simulink library "fc_vt_lib"  (Simulink 4.00)
undefined symbols (not defined in the file or in its folder): amb_tmp, compressor_mass_flow_map, compressor_pressure_map, compressor_temperature_rise_map, fc_air_comp_scale, fc_allowable_temp_rise, fc_cathode_pressure_drop, fc_cell_area, fc_cell_num, fc_comp_adeff_max, fc_comp_elec_eff, fc_comp_max_tmp, fc_comp_slpm_air_max, fc_comp_spd_max, fc_comp_voleff_max, fc_condenser_fan_flowrate, fc_condenser_fan_num, fc_condenser_fan_pwr_map, fc_condenser_frontal_area, fc_condenser_scale, fc_coolant_pump_flow_map, fc_coolant_pump_pwr_map, fc_cp_air, fc_cp_h2o_l, fc_cp_stack, fc_fuel_lhv, fc_k_air, fc_max_cathode_inlet_pressure, fc_min_cathode_inlet_pressure, fc_min_cell_volts, fc_min_sys_pwr_req, fc_min_temp_for_heat_rejection, fc_mw_air, fc_mw_h2, fc_mw_h20, fc_o2_percent, fc_p_amb, fc_polar_param_concentration, fc_polar_param_ohmic, fc_polar_param_ohmic_temp, fc_polar_param_ref_temp, fc_polar_param_tafel, fc_polar_param_temperature, fc_polar_param_voc, fc_radiator_bypass_delta_t, fc_radiator_fan_flowrate, fc_radiator_fan_num, fc_radiator_fan_pwr_map, fc_radiator_frontal_area, fc_radiator_no_fan_flowrate, fc_radiator_scale, fc_radiator_spd_ratio_fan_off, fc_radiator_spd_ratio_fan_on, fc_radiator_veh_spd_map, fc_reference_temperature, fc_rh_amb, fc_stack_i_map, fc_stack_pres_cor_map, fc_stack_pres_map, fc_stack_stoich_air_map ... (+10)
libraries: fc_vt_lib x54, simulink3 x9
(part 1 of 3)
settings Model: LastModifiedBy=kharalds

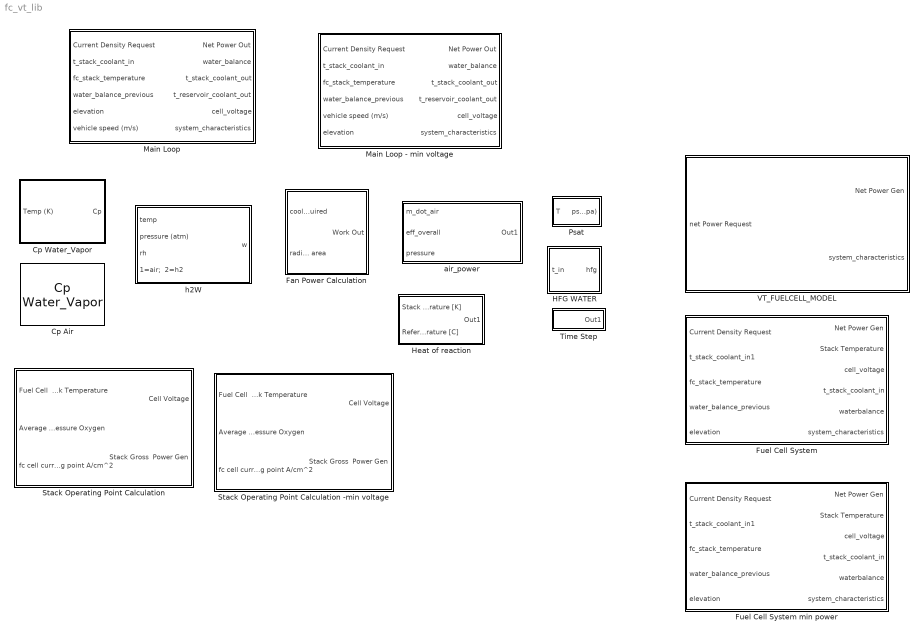
== system fc_vt_lib ==
  Cp Air : fc_vt_lib/Cp Water_Vapor
      settings: RTWFcnNameOpts=Auto  RTWFileNameOpts=Auto
  Cp Water_Vapor : Subsystem
      settings: RTWFcnNameOpts=Auto  RTWFileNameOpts=Auto
  Fan Power Calculation : Subsystem
      settings: RTWFcnNameOpts=Auto  RTWFileNameOpts=Auto
  Fuel Cell System : Subsystem
      settings: RTWFcnNameOpts=Auto  RTWFileNameOpts=Auto
  Fuel Cell System min power : Subsystem
      settings: RTWFcnNameOpts=Auto  RTWFileNameOpts=Auto
  HFG WATER : Subsystem
      settings: RTWFcnNameOpts=Auto  RTWFileNameOpts=Auto
  Heat of reaction : Subsystem
      settings: RTWFcnNameOpts=Auto  RTWFileNameOpts=Auto
  Main Loop : Subsystem
      settings: RTWFcnNameOpts=Auto  RTWFileNameOpts=Auto
  Main Loop - min voltage : Subsystem
      settings: RTWFcnNameOpts=Auto  RTWFileNameOpts=Auto
  Psat : Subsystem
      settings: RTWFcnNameOpts=Auto  RTWFileNameOpts=Auto
  Stack Operating Point Calculation : Subsystem
      settings: RTWFcnNameOpts=Auto  RTWFileNameOpts=Auto
  Stack Operating Point Calculation -min voltage : Subsystem
      settings: RTWFcnNameOpts=Auto  RTWFileNameOpts=Auto
  Time Step : Subsystem
      settings: RTWFcnNameOpts=Auto  RTWFileNameOpts=Auto
  VT_FUELCELL_MODEL : Subsystem
      settings: RTWFcnNameOpts=Auto  RTWFileNameOpts=Auto
  air_power : Subsystem
      settings: RTWFcnNameOpts=Auto  RTWFileNameOpts=Auto
  h2W : Subsystem
      settings: RTWFcnNameOpts=Auto  RTWFileNameOpts=Auto

== system fc_vt_lib/Cp Water_Vapor ==
  Temp (K) : Inport  Port=1  LatchInput=off
  A : Constant  Value=32.24
  B : Constant  Value=.1923E-2
  C : Constant  Value=1.055E-5
  D : Constant  Value=-3.595E-9
  D1 : Constant  Value=3
  D2 : Constant  Value=2
  Gain : Gain  Gain=1000  Multiplication=Element-wise(K.*u)  SaturateOnIntegerOverflow=on
  Gain1 : Gain  Gain=1/18.015  Multiplication=Element-wise(K.*u)  SaturateOnIntegerOverflow=on
  Math Function : Math  Operator=pow  OutputSignalType=auto
  Math Function1 : Math  Operator=pow  OutputSignalType=auto
  Product : Product  Inputs=2  Multiplication=Element-wise(.*)  SaturateOnIntegerOverflow=on
  Product1 : Product  Inputs=2  Multiplication=Element-wise(.*)  SaturateOnIntegerOverflow=on
  Product2 : Product  Inputs=2  Multiplication=Element-wise(.*)  SaturateOnIntegerOverflow=on
  Sum : Sum  Inputs=++++  SaturateOnIntegerOverflow=on
  Cp : Outport  Port=1
  wires:
  A/1 -> Sum/1
  B/1 -> Product/2
  Product/1 -> Sum/2
  Math Function/1 -> Product1/1
  C/1 -> Product1/2
  Math Function1/1 -> Product2/1
  D/1 -> Product2/2
  D1/1 -> Math Function1/2
  D2/1 -> Math Function/2
  Temp (K)/1 -> Math Function1/1, Math Function/1, Product/1
  Product1/1 -> Sum/3
  Product2/1 -> Sum/4
  Sum/1 -> Gain/1
  Gain/1 -> Gain1/1
  Gain1/1 -> Cp/1

== system fc_vt_lib/Fan Power Calculation ==
  cooling air  required : Inport  Port=1  LatchInput=off
  radiator frontal area : Inport  Port=2  LatchInput=off
  Constant : Constant  Value=273.15
  Constant2 : Constant  Value=fc_cp_air
  Math Function : Math  Operator=pow  OutputSignalType=auto
  Pressure Drop Relation massflow (kg/s)->Pa : Fcn  Expr=(326.21*u(1)-75.396)+101325
  Product2 : Product  Inputs=*/  Multiplication=Element-wise(.*)  SaturateOnIntegerOverflow=on
  Sum : Sum  Inputs=|++  SaturateOnIntegerOverflow=on
  Sum2 : Sum  Inputs=-+  SaturateOnIntegerOverflow=on
  Sum3 : Sum  Inputs=-+  SaturateOnIntegerOverflow=on
  T_amb1 : Constant  Value=fc_k_air
  T_amb2 : Constant  Value=1
  Work Fan  Temperature  Difference Calc1 : Product  Inputs=*/  Multiplication=Element-wise(.*)  SaturateOnIntegerOverflow=on
  Work Fan Calc : Product  Inputs=****/  Multiplication=Element-wise(.*)  SaturateOnIntegerOverflow=on
  ambient temp (C) : Constant  Value=amb_tmp
  leave it alone!4 : Constant  Value=101325
  Work Out : Outport  Port=1
  wires:
  Constant2/1 -> Work Fan Calc/3
  Sum2/1 -> Work Fan  Temperature  Difference Calc1/1
  T_amb2/1 -> Sum2/1, Sum3/1
  T_amb1/1 -> Sum2/2, Work Fan  Temperature  Difference Calc1/2
  Pressure Drop Relation massflow (kg/s)->Pa/1 -> Product2/1
  leave it alone!4/1 -> Product2/2
  Product2/1 -> Math Function/1
  cooling air  required/1 -> Work Fan Calc/2, Pressure Drop Relation massflow (kg/s)->Pa/1
  radiator frontal area/1 -> Work Fan Calc/5
  Work Fan Calc/1 -> Work Out/1
  Math Function/1 -> Sum3/2
  Work Fan  Temperature  Difference Calc1/1 -> Math Function/2
  Sum3/1 -> Work Fan Calc/1
  Sum/1 -> Work Fan Calc/4
  Constant/1 -> Sum/1
  ambient temp (C)/1 -> Sum/2

== system fc_vt_lib/Fuel Cell System ==
  " Current Density Request" : Inport  Port=1  LatchInput=off
  t_stack_coolant_in1 : Inport  Port=2  LatchInput=off
  fc_stack_temperature : Inport  Port=3  LatchInput=off
  water_balance_previous : Inport  Port=4  LatchInput=off
  elevation : Inport  Port=5  LatchInput=off
  Main Loop : fc_vt_lib/Main Loop
      settings: RTWFcnNameOpts=Auto  RTWFileNameOpts=Auto
  Net Power Gen : Outport  Port=1
  Stack Temperature : Outport  Port=2
  cell_voltage : Outport  Port=3
  t_stack_coolant_in : Outport  Port=4
  waterbalance : Outport  Port=5
  system_characteristics : Outport  Port=6
  wires:
  Main Loop/1 -> Net Power Gen/1
  Main Loop/4 -> t_stack_coolant_in/1
  Main Loop/3 -> Stack Temperature/1
  Main Loop/2 -> waterbalance/1
  " Current Density Request"/1 -> Main Loop/1
  Main Loop/5 -> cell_voltage/1
  t_stack_coolant_in1/1 -> Main Loop/2
  fc_stack_temperature/1 -> Main Loop/3
  water_balance_previous/1 -> Main Loop/4
  Main Loop/6 -> system_characteristics/1
  elevation/1 -> Main Loop/5

== system fc_vt_lib/Fuel Cell System min power ==
  Current Density Request : Inport  Port=1  LatchInput=off
  t_stack_coolant_in1 : Inport  Port=2  LatchInput=off
  fc_stack_temperature : Inport  Port=3  LatchInput=off
  water_balance_previous : Inport  Port=4  LatchInput=off
  elevation : Inport  Port=5  LatchInput=off
  Main Loop : Subsystem
      settings: RTWFcnNameOpts=Auto  RTWFileNameOpts=Auto
  Net Power Gen : Outport  Port=1
  Stack Temperature : Outport  Port=2
  cell_voltage : Outport  Port=3
  t_stack_coolant_in : Outport  Port=4
  waterbalance : Outport  Port=5
  system_characteristics : Outport  Port=6
  wires:
  water_balance_previous/1 -> Main Loop/4(water_balance_previous)
  fc_stack_temperature/1 -> Main Loop/3(fc_stack_temperature7)
  t_stack_coolant_in1/1 -> Main Loop/2(t_stack_coolant_in)
  Current Density Request/1 -> Main Loop/1(Gross Power Request)
  Main Loop/6(system_characteristics) -> system_characteristics/1
  Main Loop/5(cell_voltage) -> cell_voltage/1
  Main Loop/4(t_reservoir_coolant_out) -> t_stack_coolant_in/1
  Main Loop/3(t_stack_coolant_out) -> Stack Temperature/1
  Main Loop/2(water_balance) -> waterbalance/1
  Main Loop/1(Net Power Out) -> Net Power Gen/1
  elevation/1 -> Main Loop/5(elevation)

== system fc_vt_lib/HFG WATER ==
  t_in : Inport  Port=1  LatchInput=off
  Constant : Constant  Value=-2.4322
  Constant1 : Constant  Value=2503
  Constant2 : Constant  Value=273.15
  Gain : Gain  Gain=1000  Multiplication=Element-wise(K.*u)  SaturateOnIntegerOverflow=on
  Product : Product  Inputs=2  Multiplication=Element-wise(.*)  SaturateOnIntegerOverflow=on
  Sum : Sum  Inputs=|++  SaturateOnIntegerOverflow=on
  Sum1 : Sum  Inputs=|+-  SaturateOnIntegerOverflow=on
  hfg : Outport  Port=1
  wires:
  Gain/1 -> hfg/1
  Sum/1 -> Gain/1
  Constant1/1 -> Sum/2
  Product/1 -> Sum/1
  Constant/1 -> Product/2
  Sum1/1 -> Product/1
  Constant2/1 -> Sum1/2
  t_in/1 -> Sum1/1

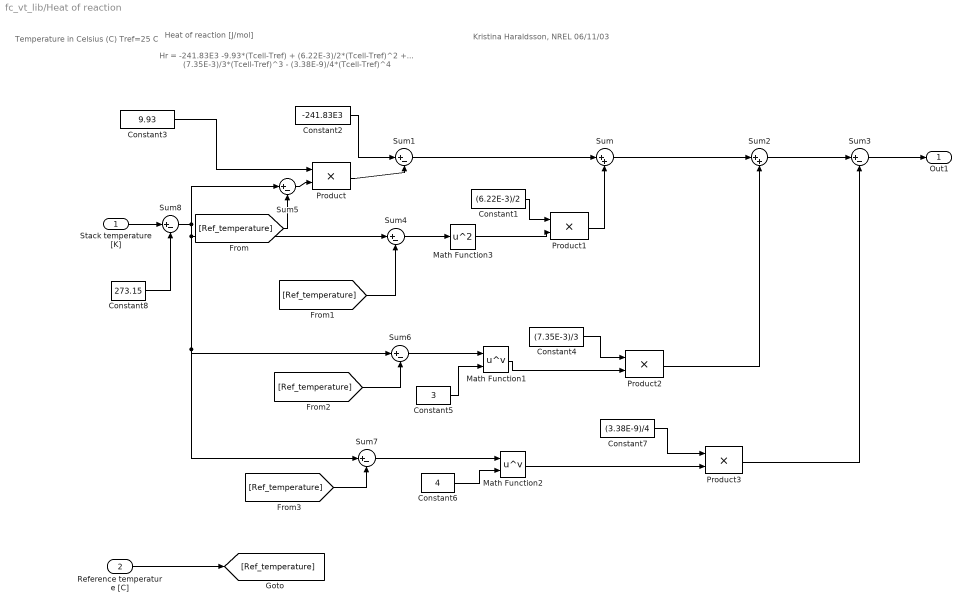
== system fc_vt_lib/Heat of reaction ==
  note: Temperature in Celsius (C)
      | Tref=25 C
  note: Hr = -241.83E3 -9.93*(Tcell-Tref) + (6.22E-3)/2*(Tcell-Tref)^2 +...
      |   (7.35E-3)/3*(Tcell-Tref)^3 - (3.38E-9)/4*(Tcell-Tref)^4
  note: Heat of reaction [J/mol]
  note: Kristina Haraldsson, NREL
      | 06/11/03
  Stack temperature [K] : Inport  Port=1  LatchInput=off
  Reference temperature [C] : Inport  Port=2  LatchInput=off
  Constant1 : Constant  Value=(6.22E-3)/2
  Constant2 : Constant  Value=-241.83E3
  Constant3 : Constant  Value=9.93
  Constant4 : Constant  Value=(7.35E-3)/3
  Constant5 : Constant  Value=3
  Constant6 : Constant  Value=4
  Constant7 : Constant  Value=(3.38E-9)/4
  Constant8 : Constant  Value=273.15
  Math Function1 : Math  Operator=pow  OutputSignalType=auto
  Math Function2 : Math  Operator=pow  OutputSignalType=auto
  Math Function3 : Math  Operator=square  OutputSignalType=auto
  Product{,1..3} (4 alike) : Product  Inputs=2  Multiplication=Element-wise(.*)  SaturateOnIntegerOverflow=on
  Sum : Sum  Inputs=|++  SaturateOnIntegerOverflow=on
  Sum{1,3..8} (7 alike) : Sum  Inputs=|+-  SaturateOnIntegerOverflow=on
  Sum2 : Sum  Inputs=|++  SaturateOnIntegerOverflow=on
  Out1 : Outport  Port=1
  wires:
  Constant3/1 -> Product/1
  Product1/1 -> Sum/2
  Product/1 -> Sum1/2
  Constant2/1 -> Sum1/1
  Sum1/1 -> Sum/1
  Sum/1 -> Sum2/1
  Constant1/1 -> Product1/1
  Math Function1/1 -> Product2/2
  Constant4/1 -> Product2/1
  Product2/1 -> Sum2/2
  Sum2/1 -> Sum3/1
  Sum3/1 -> Out1/1
  Math Function2/1 -> Product3/2
  Product3/1 -> Sum3/2
  Constant7/1 -> Product3/1
  Constant5/1 -> Math Function1/2
  Constant6/1 -> Math Function2/2
  [Ref_temperature] -> Sum4/2
  Sum5/1 -> Product/2
  Sum4/1 -> Math Function3/1
  Math Function3/1 -> Product1/2
  [Ref_temperature] -> Sum6/2
  Sum6/1 -> Math Function1/1
  [Ref_temperature] -> Sum7/2
  Sum7/1 -> Math Function2/1
  Reference temperature [C]/1 -> [Ref_temperature]
  [Ref_temperature] -> Sum5/2
  Stack temperature [K]/1 -> Sum8/1
  Sum8/1 -> Sum5/1, Sum4/1, Sum6/1, Sum7/1
  Constant8/1 -> Sum8/2

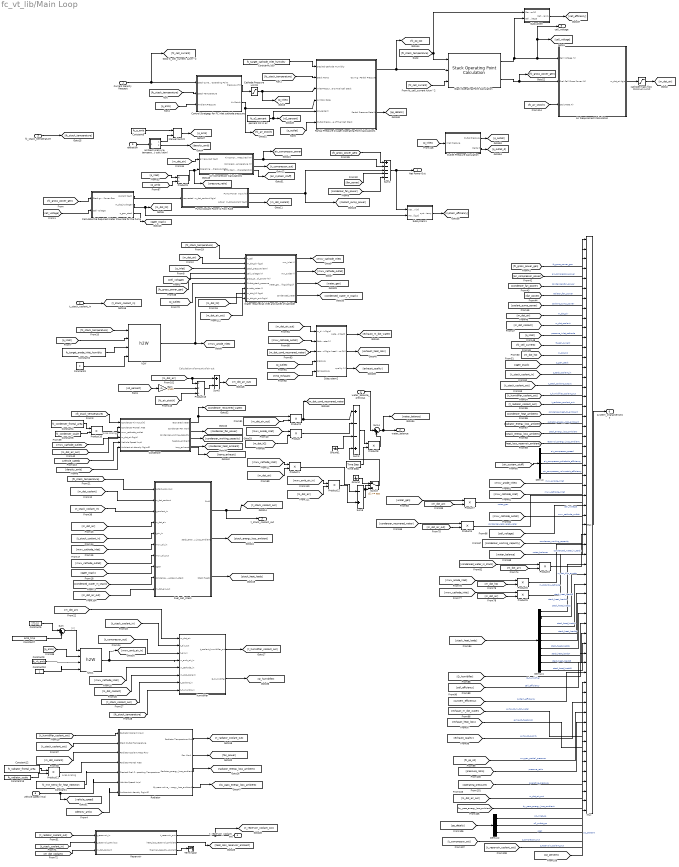
== system fc_vt_lib/Main Loop ==
  note: [K]
  note: Area scaling
  note: Area scaling
  note: Calculation of amount of air out
  Current Density Request : Inport  Port=1  LatchInput=off
  t_stack_coolant_in : Inport  Port=2  LatchInput=off
  fc_stack_temperature : Inport  Port=3  LatchInput=off
  water_balance_previous : Inport  Port=4  LatchInput=off
  elevation : Inport  Port=5  LatchInput=off
  vehicle speed (m/s) : Inport  Port=6  LatchInput=off
  Air Compressor Calculations : Subsystem
      settings: RTWFcnNameOpts=Auto  RTWFileNameOpts=Auto
  Air Requirement Calculation : Subsystem  Description=This block calculates the required amount of air needed to operate at this point.
      settings: RTWFcnNameOpts=Auto  RTWFileNameOpts=Auto
  Calculate the Required Water Flowrate for the Pump : Subsystem
      settings: RTWFcnNameOpts=Auto  RTWFileNameOpts=Auto
  "Cathode Pressure Limits " : Saturate  UpperLimit=fc_max_cathode_inlet_pressure  LowerLimit=fc_min_cathode_inlet_pressure  LinearizeAsGain=on
  Condenser : Subsystem
      settings: RTWFcnNameOpts=Auto  RTWFileNameOpts=Auto
  Constan%/100 : Constant  Value=fc_target_cathode_inlet_humidity
  Constant1 : Constant  Value=fc_min_temp_for_heat_rejection
  Constant10 : Constant  Value=1
  Constant12 : Constant  Value=fc_radiator_frontal_area
  Constant13 : Constant  Value=fc_radiator_scale
  Constant2 : Constant  Value=fc_target_anode_inlet_humidity
  Constant3 : Constant  Value=2
  Constant4 : Constant  Value=fc_condenser_frontal_area
  Constant5 : Constant  Value=273.15
  Constant6 : Constant  Value=fc_p_amb
  Constant7 : Constant  Value=amb_tmp
  Constant8 : Constant  Value=fc_condenser_scale
  Constant9 : Constant  Value=fc_rh_amb
  Control Stratgegy for FC inlet cathode pressure : Subsystem
      settings: RTWFcnNameOpts=Auto  RTWFileNameOpts=Auto
  Demux : Demux  Outputs=3  BusSelectionMode=off
  Demux1 : Demux  Outputs=9  BusSelectionMode=off
  Demux2 : Demux  Outputs=3  BusSelectionMode=off
  Fuel_cell_stack : Subsystem
      settings: RTWFcnNameOpts=Auto  RTWFileNameOpts=Auto
  Gain : Gain  Gain=1/100  Multiplication=Element-wise(K.*u)  SaturateOnIntegerOverflow=on
  Ground : Ground
  Ground1 : Ground
  Manual Switch : simulink3/Nonlinear/Manual Switch  sw=0  action=0
  Mux : Mux  Inputs=59
  Outlet Pressure Calculation : Subsystem
      settings: RTWFcnNameOpts=Auto  RTWFileNameOpts=Auto
  Partial Pressure Oxygen Operating Point Calculation1 : Subsystem
      settings: RTWFcnNameOpts=Auto  RTWFileNameOpts=Auto
  Product{,1..8,10..12} (12 alike) : Product  Inputs=2  Multiplication=Element-wise(.*)  SaturateOnIntegerOverflow=on
  Product13 : Product  Inputs=**/  Multiplication=Element-wise(.*)  SaturateOnIntegerOverflow=on
  Product9 : Product  Inputs=*/  Multiplication=Element-wise(.*)  SaturateOnIntegerOverflow=on
  Pump Coolant Power & Flow Rate : Subsystem
      settings: RTWFcnNameOpts=Auto  RTWFileNameOpts=Auto
  Radiator : Subsystem
      settings: RTWFcnNameOpts=Auto  RTWFileNameOpts=Auto
  Reservoir : Subsystem
      settings: RTWFcnNameOpts=Auto  RTWFileNameOpts=Auto
  Stack Operating Point Calculation : fc_vt_lib/Stack Operating Point Calculation
      settings: RTWFcnNameOpts=Auto  RTWFileNameOpts=Auto
  Subsystem : Subsystem
      settings: RTWFcnNameOpts=Auto  RTWFileNameOpts=Auto
  Subsystem1 : Subsystem
      settings: RTWFcnNameOpts=Auto  RTWFileNameOpts=Auto
  Subsystem2 : Subsystem
      settings: RTWFcnNameOpts=Auto  RTWFileNameOpts=Auto
  Sum : Sum  Inputs=|++  SaturateOnIntegerOverflow=on
  Sum2 : Sum  Inputs=+----  SaturateOnIntegerOverflow=on
  Sum3 : Sum  Inputs=+--+  SaturateOnIntegerOverflow=on
  Sum4 : Sum  Inputs=|++  SaturateOnIntegerOverflow=on
  Sum5 : Sum  Inputs=+-  SaturateOnIntegerOverflow=on
  Sum6 : Sum  Inputs=-+  SaturateOnIntegerOverflow=on
  Switch : Switch  Threshold=eps
  Terminator : Terminator
  Time Step : fc_vt_lib/Time Step
      settings: RTWFcnNameOpts=Auto  RTWFileNameOpts=Auto
  Water required at inlet and outlet of Cathode : Subsystem
      settings: RTWFcnNameOpts=Auto  RTWFileNameOpts=Auto
  "ambient pressure, temperature & density calc (atm)" : Subsystem
      settings: RTWFcnNameOpts=Auto  RTWFileNameOpts=Auto
  cathode mass flow Minimum Limit : Saturate  UpperLimit=1  LowerLimit=.01  LinearizeAsGain=on
  h2W : fc_vt_lib/h2W
      settings: RTWFcnNameOpts=Auto  RTWFileNameOpts=Auto
  h2W1 : fc_vt_lib/h2W
      settings: RTWFcnNameOpts=Auto  RTWFileNameOpts=Auto
  humidifier : Subsystem
      settings: RTWFcnNameOpts=Auto  RTWFileNameOpts=Auto
  percent O2 in air : Constant  Value=fc_o2_percent
  Net Power Out : Outport  Port=1
  water_balance : Outport  Port=2
  t_stack_coolant_out : Outport  Port=3
  t_reservoir_coolant_out : Outport  Port=4
  cell_voltage : Outport  Port=5
  system_characteristics : Outport  Port=6
  wires:
  [m_dot_air_out] -> Product2/2
  Product2/1 -> [m_dot_cond_recovered_water], Sum3/1
  [m_dot_air] -> Product1/2
  [mwv_cathode_inlet] -> Product1/1
  [m_dot_h2] -> Product/2
  Product/1 -> Sum3/2
  [mwv_anode_inlet] -> Product/1
  [m_dot_h2] -> Water required at inlet and outlet of Cathode/8(m_dot_h2 (kg/s))
  [condensed_water_in_stack] -> Fuel_cell_stack/9(condensed_water_in_stack)
  [cell_voltage] -> Calculate the Required Water Flowrate for the Pump/2(Cell Voltage)
  Calculate the Required Water Flowrate for the Pump/1(coolant (kg/s)) -> Pump Coolant Power & Flow Rate/1(requested  m_dot_coolant (kg/s))
  [fc_gross_power_gen] -> Calculate the Required Water Flowrate for the Pump/1(Stack gross Power Gen)
  Pump Coolant Power & Flow Rate/1(Pump Power  Input (W)) -> Sum2/3, [coolant_pump_power]
  Calculate the Required Water Flowrate for the Pump/2(m_dot_hydrogen) -> [m_dot_h2], Subsystem1/2(mass flow H2 [kg/s])
  Sum3/1 -> Product8/1
  Air Compressor Calculations/2(Compressor Outlet  Temperature (K)) -> [t_compressor_out]
  Calculate the Required Water Flowrate for the Pump/3(q_gen_stack) -> [qgen_stack]
  t_stack_coolant_in/1 -> [t_stack_coolant_in]
  [fan_power] -> Sum2/4
  [fc_stack_temperature] -> Control Stratgegy for FC inlet cathode pressure/2(Stack Temperature)
  cathode mass flow Minimum Limit/1 -> [m_dot_air]
  [m_dot_air] -> Air Compressor Calculations/1(" air required (kg/s)")
  [fc_gross_power_gen] -> Sum2/1
  fc_stack_temperature/1 -> [fc_stack_temperature]
  Pump Coolant Power & Flow Rate/2(actual  m_dot_coolant (kg/s)) -> [m_dot_coolant]
  Air Compressor Calculations/1(Air Compressor Power Required (W)) -> [air_compressor_power], Sum2/2
  [t_humidifier_coolant_out] -> Radiator/1(Radiator Coolant Input)
  [t_stack_coolant_out] -> Radiator/2(Stack Outlet Temperature)
  Radiator/1(Radiator Temperature Out) -> [t_radiator_coolant_out]
  Radiator/2(Fan Work) -> [fan_power]
  [m_dot_coolant] -> Radiator/3(Radiator Coolant Mass Flow)
  [fc_air_stoich] -> Air Requirement Calculation/3(Stoic Rate Air)
  Stack Operating Point Calculation/2 -> Air Requirement Calculation/2(Fuel Cell Gross Power (W)), [fc_gross_power_gen]
  [fc_stack_temperature] -> Subsystem/1(Stack temperature [K]), Stack Operating Point Calculation/1
  [fc_stack_temperature] -> Partial Pressure Oxygen Operating Point Calculation1/2("Stack Temp ")
  Current Density Request/1 -> [fc_cell_current], Control Stratgegy for FC inlet cathode pressure/1(Stack Current Density Operating Point)
  "Cathode Pressure Limits "/1 -> [p_inlet], Partial Pressure Oxygen Operating Point Calculation1/3(Inlet Pressure to Fuel Cell Stack)
  Control Stratgegy for FC inlet cathode pressure/1(Pressure ATM) -> "Cathode Pressure Limits "/1
  Stack Operating Point Calculation/1 -> Air Requirement Calculation/1(Cell Voltage (V)), [cell_voltage], cell_voltage/1, Subsystem/2(cell voltage)
  [fc_cell_current] -> Stack Operating Point Calculation/3
  Constan%/100/1 -> Partial Pressure Oxygen Operating Point Calculation1/1(Desired Cathode Humidity)
  Air Requirement Calculation/1(m_dot_air kg/s) -> cathode mass flow Minimum Limit/1
  Partial Pressure Oxygen Operating Point Calculation1/1(O2 Avg  Partial Pressure) -> [fc_pp_o2], Stack Operating Point Calculation/2
  Constant1/1 -> Radiator/5(Desired Fuel Cell Operating Temperature)
  [fc_stack_temperature] -> Water required at inlet and outlet of Cathode/1(T_cell)
  [m_dot_air] -> Water required at inlet and outlet of Cathode/2(m_dot_air (kg/s))
  [cell_voltage] -> Water required at inlet and outlet of Cathode/4(cell_voltage (V))
  [fc_gross_power_gen] -> Water required at inlet and outlet of Cathode/5(gross_stack_power (W))
  Water required at inlet and outlet of Cathode/1(mw_inlet (-)) -> [mwv_cathode_inlet]
  Water required at inlet and outlet of Cathode/2(mw_outlet (-)) -> [mwv_cathode_outlet]
  [fc_stack_temperature] -> h2W/1
  [p_inlet] -> h2W/2
  Constant2/1 -> h2W/3
  Constant3/1 -> h2W/4
  h2W/1 -> [mwv_anode_inlet], Water required at inlet and outlet of Cathode/7(anode_water (-))
  [p_amb] -> h2W1/2
  Constant9/1 -> h2W1/3
  Constant10/1 -> h2W1/4
  [t_radiator_coolant_out] -> Reservoir/1(t_reservoir_in)
  Reservoir/1(t_reservoir_out) -> t_reservoir_coolant_out/1, [t_reservoir_coolant_out]
  [m_dot_air] -> humidifier/1(m_dot_air)
  [t_stack_coolant_in] -> humidifier/2(t_air_out)
  [t_compressor_out] -> humidifier/3(t_air_in)
  h2W1/1 -> humidifier/4(w_amb_air_in), [mwv_amb_air_in]
  [mwv_cathode_inlet] -> humidifier/5(w_cathode_in)
  [m_dot_coolant] -> humidifier/6(m_dot_coolant)
  [t_stack_coolant_out] -> humidifier/7(t_coolant_in)
  [fc_stack_temperature] -> humidifier/8(t_hum_h20_in)
  humidifier/1(t_coolant_humidifier_out) -> [t_humidifier_coolant_out]
  [fc_stack_temperature] -> Fuel_cell_stack/1(t_stack_previous)
  [m_dot_coolant] -> Fuel_cell_stack/2(m_dot_coolant)
  [t_stack_coolant_in] -> Fuel_cell_stack/3(t_coolant_in)
  [m_dot_air] -> Fuel_cell_stack/4(m_dot_air)
  [t_stack_coolant_in] -> Fuel_cell_stack/5(t_air_in)
  [mwv_cathode_inlet] -> Fuel_cell_stack/6(mwv_air_in)
  [mwv_cathode_outlet] -> Fuel_cell_stack/7(mwv_air_out)
  [qgen_stack] -> Fuel_cell_stack/8(qgen)
  Fuel_cell_stack/1(Out1) -> [t_stack_coolant_out], t_stack_coolant_out/1
  [fc_stack_temperature] -> Condenser/1(Condenser Air Input [K])
  Condenser/1(recovered water) -> Product2/1, [condenser_recovered_water]
  Condenser/2(Condenser Fan Work) -> [condenser_fan_power]
  [mwv_cathode_outlet] -> Condenser/3(mwv_cathode_outlet)
  [m_dot_air_out] -> Condenser/4(m_dot_air [kg/s])
  Fuel_cell_stack/2(stack_energy_loss_ambient) -> [stack_energy_loss_ambient]
  Reservoir/2(heat_loss_reservoir_ambient) -> [heat_loss_reservoir_ambient]
  Radiator/3(Radiator_energy_loss_ambient) -> [radiator_energy_loss_ambient]
  [condenser_fan_power] -> Sum2/5
  Water required at inlet and outlet of Cathode/3(water_gen  ((kg/s)/(kg/s))) -> [water_gen]
  Demux/3 -> Mux/22  "air_compressor_volumetric_efficiency"
  Demux/2 -> Mux/21  "air_compressor_adiabatic_efficiency"
  Demux/1 -> Mux/20  "air_compressor_speed"
  [heat_loss_reservoir_ambient] -> Mux/19  "reservoir_energy_loss_ambient"
  [stack_energy_loss_ambient] -> Mux/18  "stack_energy_loss_ambient"
  [radiator_energy_loss_ambient] -> Mux/17  "radiator_energy_loss_ambient"
  [condenser_heat_ambient] -> Mux/16  "condenser_heat_to_ambient"
  [t_radiator_coolant_out] -> Mux/15  "t_radiator_coolant_out"
  [t_humidifier_coolant_out] -> Mux/14  "t_humidifier_coolant_out"
  [t_stack_coolant_out] -> Mux/13  "t_stack_coolant_output"
  [t_stack_coolant_in] -> Mux/12  "t_stack_coolant_in"
  [qgen_stack] -> Mux/11  "q_gen_stack"
  [m_dot_h2] -> Mux/10  "m_dot_h2"
  [fc_cell_current] -> Mux/9  "fc_cell_current"
  [p_inlet] -> Mux/8  "pressure_inlet_cathode"
  [m_dot_coolant] -> Mux/7  "m_dot_coolant"
  [m_dot_air] -> Mux/6  "m_dot_air"
  [coolant_pump_power] -> Mux/5  "coolant_pump_power"
  [fan_power] -> Mux/4  "radiator_fan_power"
  [condenser_fan_power] -> Mux/3  "condenser_fan_power"
  [air_compressor_power] -> Mux/2  "air_compressor_power"
  [fc_gross_power_gen] -> Mux/1  "fc_gross_power_gen"
  Condenser/4(heat_to_ambient) -> [condenser_heat_ambient]
  Air Compressor Calculations/3(air system  characteristics) -> [air_system_stuff]
  [air_system_stuff] -> Demux/1
  Mux/1 -> system_characteristics/1
  Product4/1 -> Mux/27  "condenser_recovered_water"
  [mwv_cathode_outlet] -> Mux/26  "mwv_cathode_outlet"
  Product7/1 -> Mux/25  "water_gen"
  [mwv_cathode_inlet] -> Mux/24  "mwv_cathode_inlet"
  [mwv_anode_inlet] -> Mux/23  "mwv_anode_inlet"
  [cell_voltage] -> Mux/28  "cell_voltage"
  Sum2/1 -> Net Power Out/1, Subsystem1/1(net power [W])
  Condenser/3(condenser_working_capacity) -> [condenser_working_capacity]
  [condenser_working_capacity] -> Mux/29  "condenser_working_capacity"
  [water_balance] -> Mux/30  "water_balance"
  [t_stack_coolant_in] -> Reservoir/2(t_reservoir_previous)
  [m_dot_coolant] -> Reservoir/3(m_dot_coolant)
  [p_inlet] -> Water required at inlet and outlet of Cathode/3(stack_pressure (atm))
  [p_outlet] -> Water required at inlet and outlet of Cathode/6(Outlet_stack_pressure)
  Water required at inlet and outlet of Cathode/4(condensed_water) -> [condensed_water_in_stack]
  Reservoir/3(thermal_capacity_coolant) -> Terminator/1
  Product3/1 -> Mux/31  "condensed_water_in_stack"
  Constant5/1 -> Sum/1
  Constant7/1 -> Sum/2
  Sum/1 -> h2W1/1
  [condensed_water_in_stack] -> Product3/1
  [m_dot_air] -> Product3/2
  [condenser_recovered_water] -> Product4/1
  [m_dot_air_out] -> Product4/2
  [mwv_cathode_inlet] -> Product5/1
  [m_dot_air] -> Product5/2
  [mwv_anode_inlet] -> Product6/1
  [m_dot_h2] -> Product6/2
  Product6/1 -> Mux/32  "m_dot_h2o_anode"
  Product5/1 -> Mux/33  "m_dot_h2o_cathode"
  [water_gen] -> Product7/1
  [m_dot_air] -> Product7/2
  Sum4/1 -> water_balance/1, [water_balance]
  Fuel_cell_stack/3(Stack Heats) -> [stack_heat_loads]
  [stack_heat_loads] -> Demux1/1
  Demux1/1 -> Mux/34  "stack_heat_loads1"
  Demux1/2 -> Mux/35  "stack_heat_loads2"
  Demux1/3 -> Mux/36  "stack_heat_loads3"
  Demux1/4 -> Mux/37  "stack_heat_loads4"
  Demux1/5 -> Mux/38  "stack_heat_loads5"
  Demux1/6 -> Mux/39  "stack_heat_loads6"
  Demux1/7 -> Mux/40  "stack_heat_loads7"
  Demux1/8 -> Mux/41  "stack_heat_loads8"
  Demux1/9 -> Mux/42  "stack_heat_loads9"
  water_balance_previous/1 -> Sum4/1
  Time Step/1 -> Product8/2
  Product8/1 -> Sum4/2
  Manual Switch/1 -> [p_amb]
  Constant6/1 -> Manual Switch/1
  "ambient pressure, temperature & density calc (atm)"/1("Ambient pressure [atm] ") -> Manual Switch/2
  elevation/1 -> "ambient pressure, temperature & density calc (atm)"/1(elevation)
  [p_inlet] -> Product9/1
  [p_amb] -> Product9/2
  Product9/1 -> Air Compressor Calculations/2(Operating  Pressure Ratio), [pressure_ratio]
  humidifier/2(Q_humidifier) -> [Q_humidifier]
  [Q_humidifier] -> Mux/43  "Q_humidifier"
  Constant8/1 -> Product10/2
  Constant4/1 -> Product10/1
  Product10/1 -> Condenser/2(Condenser Frontal Area)
  Constant12/1 -> Product11/1
  Constant13/1 -> Product11/2
  Product11/1 -> Radiator/4(Radiator Frontal Area)
  Subsystem/1(Cell efficiency) -> [cell_efficiency]
  [cell_efficiency] -> Mux/44  "cell_efficiency"
  Subsystem1/1("system_efficiency ") -> [system_efficiency]
  [system_efficiency] -> Mux/45  "system_efficiency"
  Subsystem2/3(quality [-]) -> [exhaust_quality]
  Subsystem2/2(heat loss [W]) -> [exhaust_heat_loss]
  Subsystem2/1(water loss [kg/s]) -> [exhaust_m_dot_water]
  Condenser/5(tmp_exhaust) -> [temp_exhaust]
  [m_dot_cond_recovered_water] -> Subsystem2/3(recovered [kg/s-)
  [m_dot_air_out] -> Subsystem2/1(m_dot_air [kg/s])
  [mwv_cathode_outlet] -> Subsystem2/2(Cathode outlet water [-])
  [p_outlet] -> Subsystem2/4(pressure)
  [tmp_exhaust] -> Subsystem2/5(temperature)
  [exhaust_quality] -> Mux/48  "exhaust_quality"
  [exhaust_heat_loss] -> Mux/47  "exhaust_heat_loss"
  [exhaust_m_dot_water] -> Mux/46  "exhaust_m_dot_water"
  [fc_pp_o2] -> Mux/49  "oxygen_partial_pressure"
  [pressure_ratio] -> Mux/50  "pressure_ratio"
  [operating_pressure] -> Mux/51  "operating_pressure"
  [o2_percent] -> Gain/1
  [fc_air_stoich] -> Product13/3
  [m_dot_air] -> Product13/1, Sum5/1
  [m_dot_air_out] -> Mux/52  "m_dot_air_out"
  [m_dot_air_out] -> Fuel_cell_stack/10(m_dot_air_out)
  Radiator/4(By-pass valve_energy_loss_ambient1) -> [by_pass_energy_loss_ambient]
  [by_pass_energy_loss_ambient] -> Mux/53  "by_pass_energy_loss_ambient"
  Product13/1 -> Sum5/2
  Sum5/1 -> [m_dot_air_out]
  Gain/1 -> Product13/2
  Partial Pressure Oxygen Operating Point Calculation1/2(Partial Pressure Details) -> [pp_details]
  [pp_details] -> Demux2/1
  Demux2/1 -> Mux/54  "o2_inlet_pp"
  Demux2/2 -> Mux/55  "o2_outlet_pp"
  Demux2/3 -> Mux/56  "psat"
  [t_compressor_out] -> Mux/57  "t_compressor_out"
  [t_reservoir_coolant_out] -> Mux/58  "t_reservoir_coolant_out"
  [o2_percent] -> Mux/59  "o2_percent"
  percent O2 in air/1 -> [o2_percent], Partial Pressure Oxygen Operating Point Calculation1/5(o2_percent)
  [m_dot_air] -> Product12/2
  [mwv_amb_air_in] -> Product12/1
  [m_dot_air_out] -> Water required at inlet and outlet of Cathode/9(m_dot_air_out (kg/s))
  vehicle speed (m/s)/1 -> Radiator/6(Vehicle Speed (m/s)), [vehicle_speed]
  [vehicle_speed] -> Condenser/5(Vehicle Speed (m/s))
  [p_amb] -> Control Stratgegy for FC inlet cathode pressure/3(Ambient Pressure)
  Sum6/1 -> Switch/2, Switch/3
  Ground/1 -> Switch/1
  Product12/1 -> Sum6/2
  Product1/1 -> Sum6/1
  Switch/1 -> Sum3/4
  Ground1/1 -> Sum3/3
  Control Stratgegy for FC inlet cathode pressure/2(Air Stoich) -> [fc_air_stoich], Partial Pressure Oxygen Operating Point Calculation1/4(Air Stoic Rate)
  Outlet Pressure Calculation/2(Delta P) -> [p_outlet_d]
  [p_inlet] -> Outlet Pressure Calculation/1(Inlet Pressure)
  Outlet Pressure Calculation/1(Outlet Pressure) -> [p_outlet]
  [p_outlet] -> Partial Pressure Oxygen Operating Point Calculation1/6(Outlet Pressure of Fuel Cell Stack)
  "ambient pressure, temperature & density calc (atm)"/2(Air density [kg/m3]) -> [density_amb]
  [density_amb] -> Radiator/7(Ambient air density [kg/m3])
  [density_amb] -> Condenser/6(Ambient air density [kg/m3])

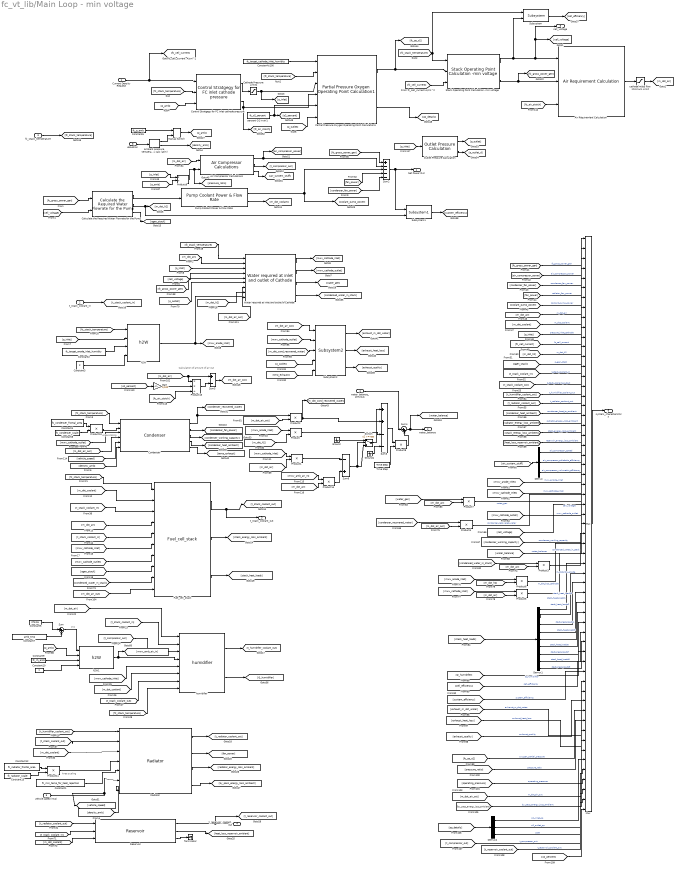
== system fc_vt_lib/Main Loop - min voltage ==
  note: [K]
  note: Area scaling
  note: Area scaling
  note: Calculation of amount of air out
  Current Density Request : Inport  Port=1  LatchInput=off
  t_stack_coolant_in : Inport  Port=2  LatchInput=off
  fc_stack_temperature : Inport  Port=3  LatchInput=off
  water_balance_previous : Inport  Port=4  LatchInput=off
  vehicle speed (m/s) : Inport  Port=5  LatchInput=off
  elevation : Inport  Port=6  LatchInput=off
  Air Compressor Calculations : fc_vt_lib/Main Loop/Air Compressor Calculations
      settings: RTWFcnNameOpts=Auto  RTWFileNameOpts=Auto
  Air Requirement Calculation : fc_vt_lib/Main Loop/Air Requirement Calculation  Description=This block calculates the required amount of air needed to operate at this point.
      settings: RTWFcnNameOpts=Auto  RTWFileNameOpts=Auto
  Calculate the Required Water Flowrate for the Pump : fc_vt_lib/Main Loop/Calculate the Required Water Flowrate for the Pump
      settings: RTWFcnNameOpts=Auto  RTWFileNameOpts=Auto
  "Cathode Pressure Limits " : Saturate  UpperLimit=fc_max_cathode_inlet_pressure  LowerLimit=fc_min_cathode_inlet_pressure  LinearizeAsGain=on
  Condenser : fc_vt_lib/Main Loop/Condenser
      settings: RTWFcnNameOpts=Auto  RTWFileNameOpts=Auto
  Constan%/100 : Constant  Value=fc_target_cathode_inlet_humidity
  Constant1 : Constant  Value=fc_min_temp_for_heat_rejection
  Constant10 : Constant  Value=1
  Constant12 : Constant  Value=fc_radiator_frontal_area
  Constant13 : Constant  Value=fc_radiator_scale
  Constant2 : Constant  Value=fc_target_anode_inlet_humidity
  Constant3 : Constant  Value=2
  Constant4 : Constant  Value=fc_condenser_frontal_area
  Constant5 : Constant  Value=273.15
  Constant6 : Constant  Value=fc_p_amb
  Constant7 : Constant  Value=amb_tmp
  Constant8 : Constant  Value=fc_condenser_scale
  Constant9 : Constant  Value=fc_rh_amb
  Control Stratgegy for FC inlet cathode pressure : fc_vt_lib/Main Loop/Control Stratgegy for FC inlet cathode pressure
      settings: RTWFcnNameOpts=Auto  RTWFileNameOpts=Auto
  Demux : Demux  Outputs=3  BusSelectionMode=off
  Demux1 : Demux  Outputs=9  BusSelectionMode=off
  Demux2 : Demux  Outputs=3  BusSelectionMode=off
  Fuel_cell_stack : fc_vt_lib/Main Loop/Fuel_cell_stack
      settings: RTWFcnNameOpts=Auto  RTWFileNameOpts=Auto
  Gain : Gain  Gain=1/100  Multiplication=Element-wise(K.*u)  SaturateOnIntegerOverflow=on
  Ground : Ground
  Ground1 : Ground
  Manual Switch : simulink3/Nonlinear/Manual Switch  sw=0  action=0
  Mux : Mux  Inputs=59
  Outlet Pressure Calculation : fc_vt_lib/Main Loop/Outlet Pressure Calculation
      settings: RTWFcnNameOpts=Auto  RTWFileNameOpts=Auto
  Partial Pressure Oxygen Operating Point Calculation1 : fc_vt_lib/Main Loop/Partial Pressure Oxygen Operating Point Calculation1
      settings: RTWFcnNameOpts=Auto  RTWFileNameOpts=Auto
  Product{,1..8,10..11,14} (12 alike) : Product  Inputs=2  Multiplication=Element-wise(.*)  SaturateOnIntegerOverflow=on
  Product13 : Product  Inputs=**/  Multiplication=Element-wise(.*)  SaturateOnIntegerOverflow=on
  Product9 : Product  Inputs=*/  Multiplication=Element-wise(.*)  SaturateOnIntegerOverflow=on
  Pump Coolant Power & Flow Rate : fc_vt_lib/Main Loop/Pump Coolant Power & Flow Rate
      settings: RTWFcnNameOpts=Auto  RTWFileNameOpts=Auto
  Radiator : fc_vt_lib/Main Loop/Radiator
      settings: RTWFcnNameOpts=Auto  RTWFileNameOpts=Auto
  Reservoir : fc_vt_lib/Main Loop/Reservoir
      settings: RTWFcnNameOpts=Auto  RTWFileNameOpts=Auto
  Stack Operating Point Calculation -min voltage : fc_vt_lib/Stack Operating Point Calculation -min voltage
      settings: RTWFcnNameOpts=Auto  RTWFileNameOpts=Auto
  Subsystem : fc_vt_lib/Main Loop/Subsystem
      settings: RTWFcnNameOpts=Auto  RTWFileNameOpts=Auto
  Subsystem1 : fc_vt_lib/Main Loop/Subsystem1
      settings: RTWFcnNameOpts=Auto  RTWFileNameOpts=Auto
  Subsystem2 : fc_vt_lib/Main Loop/Subsystem2
      settings: RTWFcnNameOpts=Auto  RTWFileNameOpts=Auto
  Sum : Sum  Inputs=|++  SaturateOnIntegerOverflow=on
  Sum2 : Sum  Inputs=+----  SaturateOnIntegerOverflow=on
  Sum3 : Sum  Inputs=++--  SaturateOnIntegerOverflow=on
  Sum4 : Sum  Inputs=|++  SaturateOnIntegerOverflow=on
  Sum5 : Sum  Inputs=+-  SaturateOnIntegerOverflow=on
  Sum6 : Sum  Inputs=-+  SaturateOnIntegerOverflow=on
  Switch : Switch  Threshold=eps
  Terminator : Terminator
  Time Step : fc_vt_lib/Time Step
      settings: RTWFcnNameOpts=Auto  RTWFileNameOpts=Auto
  Water required at inlet and outlet of Cathode : fc_vt_lib/Main Loop/Water required at inlet and outlet of Cathode
      settings: RTWFcnNameOpts=Auto  RTWFileNameOpts=Auto
  "ambient pressure, temperature & density calc (atm)" : fc_vt_lib/Main Loop/ambient pressure, temperature & density calc (atm)
      settings: RTWFcnNameOpts=Auto  RTWFileNameOpts=Auto
  cathode mass flow Minimum Limit : Saturate  UpperLimit=1  LowerLimit=.01  LinearizeAsGain=on
  h2W : fc_vt_lib/h2W
      settings: RTWFcnNameOpts=Auto  RTWFileNameOpts=Auto
  h2W1 : fc_vt_lib/h2W
      settings: RTWFcnNameOpts=Auto  RTWFileNameOpts=Auto
  humidifier : fc_vt_lib/Main Loop/humidifier
      settings: RTWFcnNameOpts=Auto  RTWFileNameOpts=Auto
  percent O2 in air1 : Constant  Value=fc_o2_percent
  Net Power Out : Outport  Port=1
  water_balance : Outport  Port=2
  t_stack_coolant_out : Outport  Port=3
  t_reservoir_coolant_out : Outport  Port=4
  cell_voltage : Outport  Port=5
  system_characteristics : Outport  Port=6
  wires:
  [m_dot_air_out] -> Product2/2
  Product2/1 -> Sum3/2, [m_dot_cond_recovered_water]
  [m_dot_air] -> Product1/2
  [mwv_cathode_inlet] -> Product1/1
  [m_dot_h2] -> Product/2
  Product/1 -> Sum3/3
  [mwv_anode_inlet] -> Product/1
  [m_dot_h2] -> Water required at inlet and outlet of Cathode/8
  [condensed_water_in_stack] -> Fuel_cell_stack/9
  [cell_voltage] -> Calculate the Required Water Flowrate for the Pump/2
  Calculate the Required Water Flowrate for the Pump/1 -> Pump Coolant Power & Flow Rate/1
  [fc_gross_power_gen] -> Calculate the Required Water Flowrate for the Pump/1
  Pump Coolant Power & Flow Rate/1 -> Sum2/3, [coolant_pump_power]
  Calculate the Required Water Flowrate for the Pump/2 -> [m_dot_h2], Subsystem1/2
  Sum3/1 -> Product8/1
  Air Compressor Calculations/2 -> [t_compressor_out]
  Calculate the Required Water Flowrate for the Pump/3 -> [qgen_stack]
  t_stack_coolant_in/1 -> [t_stack_coolant_in]
  [fan_power] -> Sum2/4
  [fc_stack_temperature] -> Control Stratgegy for FC inlet cathode pressure/2
  cathode mass flow Minimum Limit/1 -> [m_dot_air]
  [m_dot_air] -> Air Compressor Calculations/1
  [fc_gross_power_gen] -> Sum2/1
  fc_stack_temperature/1 -> [fc_stack_temperature]
  Pump Coolant Power & Flow Rate/2 -> [m_dot_coolant]
  Air Compressor Calculations/1 -> [air_compressor_power], Sum2/2
  [t_humidifier_coolant_out] -> Radiator/1
  [t_stack_coolant_out] -> Radiator/2
  Radiator/1 -> [t_radiator_coolant_out]
  Radiator/2 -> [fan_power]
  [m_dot_coolant] -> Radiator/3
  Stack Operating Point Calculation -min voltage/2 -> Air Requirement Calculation/2, [fc_gross_power_gen]
  [fc_stack_temperature] -> Subsystem/1, Stack Operating Point Calculation -min voltage/1
  [fc_stack_temperature] -> Partial Pressure Oxygen Operating Point Calculation1/2
  Current Density Request/1 -> [fc_cell_current], Control Stratgegy for FC inlet cathode pressure/1
  "Cathode Pressure Limits "/1 -> [p_inlet], Partial Pressure Oxygen Operating Point Calculation1/3
  Control Stratgegy for FC inlet cathode pressure/1 -> "Cathode Pressure Limits "/1
  Stack Operating Point Calculation -min voltage/1 -> Air Requirement Calculation/1, [cell_voltage], cell_voltage/1, Subsystem/2
  [fc_cell_current] -> Stack Operating Point Calculation -min voltage/3
  Constan%/100/1 -> Partial Pressure Oxygen Operating Point Calculation1/1
  Air Requirement Calculation/1 -> cathode mass flow Minimum Limit/1
  Partial Pressure Oxygen Operating Point Calculation1/1 -> [fc_pp_o2], Stack Operating Point Calculation -min voltage/2
  [fc_stack_temperature] -> Water required at inlet and outlet of Cathode/1
  [m_dot_air] -> Water required at inlet and outlet of Cathode/2
  [cell_voltage] -> Water required at inlet and outlet of Cathode/4
  [fc_gross_power_gen] -> Water required at inlet and outlet of Cathode/5
  Water required at inlet and outlet of Cathode/1 -> [mwv_cathode_inlet]
  Water required at inlet and outlet of Cathode/2 -> [mwv_cathode_outlet]
  [fc_stack_temperature] -> h2W/1
  [p_inlet] -> h2W/2
  Constant2/1 -> h2W/3
  Constant3/1 -> h2W/4
  h2W/1 -> [mwv_anode_inlet], Water required at inlet and outlet of Cathode/7
  [p_amb] -> h2W1/2
  Constant9/1 -> h2W1/3
  Constant10/1 -> h2W1/4
  [t_radiator_coolant_out] -> Reservoir/1
  Reservoir/1 -> t_reservoir_coolant_out/1, [t_reservoir_coolant_out]
  [m_dot_air] -> humidifier/1
  [t_stack_coolant_in] -> humidifier/2
  [t_compressor_out] -> humidifier/3
  h2W1/1 -> humidifier/4, [mwv_amb_air_in]
  [mwv_cathode_inlet] -> humidifier/5
  [m_dot_coolant] -> humidifier/6
  [t_stack_coolant_out] -> humidifier/7
  [fc_stack_temperature] -> humidifier/8
  humidifier/1 -> [t_humidifier_coolant_out]
  [fc_stack_temperature] -> Fuel_cell_stack/1
  [m_dot_coolant] -> Fuel_cell_stack/2
  [t_stack_coolant_in] -> Fuel_cell_stack/3
  [m_dot_air] -> Fuel_cell_stack/4
  [t_stack_coolant_in] -> Fuel_cell_stack/5
  [mwv_cathode_inlet] -> Fuel_cell_stack/6
  [mwv_cathode_outlet] -> Fuel_cell_stack/7
  [qgen_stack] -> Fuel_cell_stack/8
  Fuel_cell_stack/1 -> [t_stack_coolant_out], t_stack_coolant_out/1
  [fc_stack_temperature] -> Condenser/1
  Condenser/1 -> Product2/1, [condenser_recovered_water]
  Condenser/2 -> [condenser_fan_power]
  [mwv_cathode_outlet] -> Condenser/3
  [m_dot_air_out] -> Condenser/4
  Fuel_cell_stack/2 -> [stack_energy_loss_ambient]
  Reservoir/2 -> [heat_loss_reservoir_ambient]
  Radiator/3 -> [radiator_energy_loss_ambient]
  [condenser_fan_power] -> Sum2/5
  Water required at inlet and outlet of Cathode/3 -> [water_gen]
  Demux/3 -> Mux/22  "air_compressor_volumetric_efficiency"
  Demux/2 -> Mux/21  "air_compressor_adiabatic_efficiency"
  Demux/1 -> Mux/20  "air_compressor_speed"
  [heat_loss_reservoir_ambient] -> Mux/19  "reservoir_energy_loss_ambient"
  [stack_energy_loss_ambient] -> Mux/18  "stack_energy_loss_ambient"
  [radiator_energy_loss_ambient] -> Mux/17  "radiator_energy_loss_ambient"
  [condenser_heat_ambient] -> Mux/16  "condenser_heat_to_ambient"
  [t_radiator_coolant_out] -> Mux/15  "t_radiator_coolant_out"
  [t_humidifier_coolant_out] -> Mux/14  "t_humidifier_coolant_out"
  [t_stack_coolant_out] -> Mux/13  "t_stack_coolant_output"
  [t_stack_coolant_in] -> Mux/12  "t_stack_coolant_in"
  [qgen_stack] -> Mux/11  "q_gen_stack"
  [m_dot_h2] -> Mux/10  "m_dot_h2"
  [fc_cell_current] -> Mux/9  "fc_cell_current"
  [p_inlet] -> Mux/8  "pressure_inlet_cathode"
  [m_dot_coolant] -> Mux/7  "m_dot_coolant"
  [m_dot_air] -> Mux/6  "m_dot_air"
  [coolant_pump_power] -> Mux/5  "coolant_pump_power"
  [fan_power] -> Mux/4  "radiator_fan_power"
  [condenser_fan_power] -> Mux/3  "condenser_fan_power"
  [air_compressor_power] -> Mux/2  "air_compressor_power"
  [fc_gross_power_gen] -> Mux/1  "fc_gross_power_gen"
  Condenser/4 -> [condenser_heat_ambient]
  Air Compressor Calculations/3 -> [air_system_stuff]
  [air_system_stuff] -> Demux/1
  Mux/1 -> system_characteristics/1
  Product4/1 -> Mux/27  "condenser_recovered_water"
  [mwv_cathode_outlet] -> Mux/26  "mwv_cathode_outlet"
  Product7/1 -> Mux/25  "water_gen"
  [mwv_cathode_inlet] -> Mux/24  "mwv_cathode_inlet"
  [mwv_anode_inlet] -> Mux/23  "mwv_anode_inlet"
  [cell_voltage] -> Mux/28  "cell_voltage"
  Sum2/1 -> Net Power Out/1, Subsystem1/1
  Condenser/3 -> [condenser_working_capacity]
  [condenser_working_capacity] -> Mux/29  "condenser_working_capacity"
  [water_balance] -> Mux/30  "water_balance"
  [t_stack_coolant_in] -> Reservoir/2
  [m_dot_coolant] -> Reservoir/3
  [p_inlet] -> Water required at inlet and outlet of Cathode/3
  [p_outlet] -> Water required at inlet and outlet of Cathode/6
  Water required at inlet and outlet of Cathode/4 -> [condensed_water_in_stack]
  Reservoir/3 -> Terminator/1
  Product3/1 -> Mux/31  "condensed_water_in_stack"
  Constant5/1 -> Sum/1
  Constant7/1 -> Sum/2
  Sum/1 -> h2W1/1
  [condensed_water_in_stack] -> Product3/1
  [m_dot_air] -> Product3/2
  [condenser_recovered_water] -> Product4/1
  [m_dot_air_out] -> Product4/2
  [mwv_cathode_inlet] -> Product5/1
  [m_dot_air] -> Product5/2
  [mwv_anode_inlet] -> Product6/1
  [m_dot_h2] -> Product6/2
  Product6/1 -> Mux/32  "m_dot_h2o_anode"
  Product5/1 -> Mux/33  "m_dot_h2o_cathode"
  [water_gen] -> Product7/1
  [m_dot_air] -> Product7/2
  Sum4/1 -> water_balance/1, [water_balance]
  Fuel_cell_stack/3 -> [stack_heat_loads]
  [stack_heat_loads] -> Demux1/1
  Demux1/1 -> Mux/34  "stack_heat_loads1"
  Demux1/2 -> Mux/35  "stack_heat_loads2"
  Demux1/3 -> Mux/36  "stack_heat_loads3"
  Demux1/4 -> Mux/37  "stack_heat_loads4"
  Demux1/5 -> Mux/38  "stack_heat_loads5"
  Demux1/6 -> Mux/39  "stack_heat_loads6"
  Demux1/7 -> Mux/40  "stack_heat_loads7"
  Demux1/8 -> Mux/41  "stack_heat_loads8"
  Demux1/9 -> Mux/42  "stack_heat_loads9"
  water_balance_previous/1 -> Sum4/1
  Time Step/1 -> Product8/2
  Product8/1 -> Sum4/2
  [p_inlet] -> Product9/1
  [p_amb] -> Product9/2
  Product9/1 -> Air Compressor Calculations/2, [pressure_ratio]
  humidifier/2 -> [Q_humidifier]
  [Q_humidifier] -> Mux/43  "Q_humidifier"
  Constant8/1 -> Product10/2
  Constant4/1 -> Product10/1
  Product10/1 -> Condenser/2
  Constant12/1 -> Product11/1
  Constant13/1 -> Product11/2
  Product11/1 -> Radiator/4
  Subsystem/1 -> [cell_efficiency]
  [cell_efficiency] -> Mux/44  "cell_efficiency"
  Subsystem1/1 -> [system_efficiency]
  [system_efficiency] -> Mux/45  "system_efficiency"
  Subsystem2/3 -> [exhaust_quality]
  Subsystem2/2 -> [exhaust_heat_loss]
  Subsystem2/1 -> [exhaust_m_dot_water]
  Condenser/5 -> [temp_exhaust]
  [m_dot_cond_recovered_water] -> Subsystem2/3
  [m_dot_air_out] -> Subsystem2/1
  [mwv_cathode_outlet] -> Subsystem2/2
  [p_outlet] -> Subsystem2/4
  [tmp_exhaust] -> Subsystem2/5
  [exhaust_quality] -> Mux/48  "exhaust_quality"
  [exhaust_heat_loss] -> Mux/47  "exhaust_heat_loss"
  [exhaust_m_dot_water] -> Mux/46  "exhaust_m_dot_water"
  [fc_pp_o2] -> Mux/49  "oxygen_partial_pressure"
  [pressure_ratio] -> Mux/50  "pressure_ratio"
  [operating_pressure] -> Mux/51  "operating_pressure"
  [m_dot_air_out] -> Mux/52  "m_dot_air_out"
  [m_dot_air_out] -> Fuel_cell_stack/10
  Radiator/4 -> [by_pass_energy_loss_ambient]
  [by_pass_energy_loss_ambient] -> Mux/53  "by_pass_energy_loss_ambient"
  [o2_percent] -> Gain/1
  [m_dot_air] -> Product13/1, Sum5/1
  Product13/1 -> Sum5/2
  Sum5/1 -> [m_dot_air_out]
  Gain/1 -> Product13/2
  [pp_details] -> Demux2/1
  Demux2/2 -> Mux/55  "o2_outlet_pp"
  Demux2/3 -> Mux/56  "psat"
  [t_compressor_out] -> Mux/57  "t_compressor_out"
  [t_reservoir_coolant_out] -> Mux/58  "t_reservoir_coolant_out"
  Demux2/1 -> Mux/54  "o2_inlet_pp"
  [o2_percent] -> Mux/59
  percent O2 in air1/1 -> [o2_percent], Partial Pressure Oxygen Operating Point Calculation1/5
  Partial Pressure Oxygen Operating Point Calculation1/2 -> [pp_details]
  [m_dot_air_out] -> Water required at inlet and outlet of Cathode/9
  vehicle speed (m/s)/1 -> Radiator/6, [vehicle_speed]
  [vehicle_speed] -> Condenser/5
  [p_amb] -> Control Stratgegy for FC inlet cathode pressure/3
  [m_dot_air] -> Product14/2
  [mwv_amb_air_in] -> Product14/1
  Sum6/1 -> Switch/2, Switch/3
  Ground/1 -> Switch/1
  Product14/1 -> Sum6/2
  Product1/1 -> Sum6/1
  Switch/1 -> Sum3/1
  Ground1/1 -> Sum3/4
  Control Stratgegy for FC inlet cathode pressure/2 -> [fc_air_stoich], Partial Pressure Oxygen Operating Point Calculation1/4
  [fc_air_stoich] -> Air Requirement Calculation/3
  [fc_air_stoich] -> Product13/3
  [p_outlet] -> Partial Pressure Oxygen Operating Point Calculation1/6
  Outlet Pressure Calculation/2 -> [p_outlet_d]
  [p_inlet] -> Outlet Pressure Calculation/1
  Outlet Pressure Calculation/1 -> [p_outlet]
  Manual Switch/1 -> [p_amb]
  Constant6/1 -> Manual Switch/1
  "ambient pressure, temperature & density calc (atm)"/1 -> Manual Switch/2
  elevation/1 -> "ambient pressure, temperature & density calc (atm)"/1
  "ambient pressure, temperature & density calc (atm)"/2 -> [density_amb]
  Constant1/1 -> Radiator/5
  [density_amb] -> Radiator/7
  [density_amb] -> Condenser/6

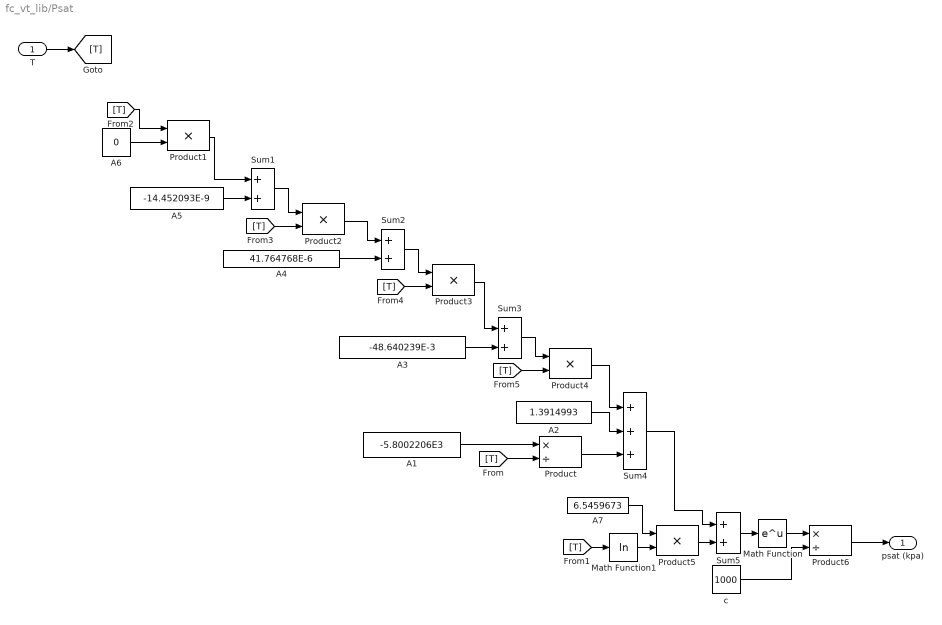
== system fc_vt_lib/Psat ==
  T : Inport  Port=1  LatchInput=off
  A1 : Constant  Value=-5.8002206E3
  A2 : Constant  Value=1.3914993
  A3 : Constant  Value=-48.640239E-3
  A4 : Constant  Value=41.764768E-6
  A5 : Constant  Value=-14.452093E-9
  A6 : Constant  Value=0
  A7 : Constant  Value=6.5459673
  Math Function : Math  Operator=exp  OutputSignalType=auto
  Math Function1 : Math  Operator=log  OutputSignalType=auto
  Product : Product  Inputs=*/  Multiplication=Element-wise(.*)  SaturateOnIntegerOverflow=on
  Product{1..5} (5 alike) : Product  Inputs=**  Multiplication=Element-wise(.*)  SaturateOnIntegerOverflow=on
  Product6 : Product  Inputs=*/  Multiplication=Element-wise(.*)  SaturateOnIntegerOverflow=on
  Sum{1..3,5} (4 alike) : Sum  Inputs=++  SaturateOnIntegerOverflow=on
  Sum4 : Sum  Inputs=+++  SaturateOnIntegerOverflow=on
  c : Constant  Value=1000
  psat (kpa) : Outport  Port=1
  wires:
  T/1 -> [T]
  A1/1 -> Product/1
  [T] -> Product/2
  [T] -> Product1/1
  A6/1 -> Product1/2
  Product1/1 -> Sum1/1
  A5/1 -> Sum1/2
  Sum1/1 -> Product2/1
  [T] -> Product2/2
  Product2/1 -> Sum2/1
  A4/1 -> Sum2/2
  Sum2/1 -> Product3/1
  [T] -> Product3/2
  Product3/1 -> Sum3/1
  A3/1 -> Sum3/2
  Sum3/1 -> Product4/1
  [T] -> Product4/2
  Product4/1 -> Sum4/1
  A2/1 -> Sum4/2
  Product/1 -> Sum4/3
  [T] -> Math Function1/1
  Math Function1/1 -> Product5/2
  A7/1 -> Product5/1
  Product5/1 -> Sum5/2
  Product6/1 -> psat (kpa)/1
  c/1 -> Product6/2
  Sum4/1 -> Sum5/1
  Sum5/1 -> Math Function/1
  Math Function/1 -> Product6/1

== system fc_vt_lib/Stack Operating Point Calculation ==
  Fuel Cell  Stack Temperature : Inport  Port=1  LatchInput=off
  Average Partial Pressure Oxygen : Inport  Port=2  LatchInput=off
  fc cell current density operating point A/cm^2 : Inport  Port=3  LatchInput=off
  Cell Gross Power Gen W/cm^2 : simulink3/Math/Dot Product
  Polarization Curve : Subsystem
      settings: RTWFcnNameOpts=Auto  RTWFileNameOpts=Auto
  Stack Gross Power Gen W1 : simulink3/Math/Dot Product
  stack area cm^2 : Constant  Value=fc_cell_area*fc_cell_num
  Cell Voltage : Outport  Port=1
  Stack Gross  Power Gen : Outport  Port=2
  wires:
  Cell Gross Power Gen W/cm^2/1 -> Stack Gross Power Gen W1/1
  stack area cm^2/1 -> Stack Gross Power Gen W1/2
  Stack Gross Power Gen W1/1 -> Stack Gross  Power Gen/1
  fc cell current density operating point A/cm^2/1 -> Cell Gross Power Gen W/cm^2/2, Polarization Curve/3(current)
  Fuel Cell  Stack Temperature/1 -> Polarization Curve/1(temperature)
  Average Partial Pressure Oxygen/1 -> Polarization Curve/2(po2)
  Polarization Curve/1(cell voltage) -> Cell Gross Power Gen W/cm^2/1, Cell Voltage/1

== system fc_vt_lib/Stack Operating Point Calculation -min voltage ==
  Fuel Cell  Stack Temperature : Inport  Port=1  LatchInput=off
  Average Partial Pressure Oxygen : Inport  Port=2  LatchInput=off
  fc cell current density operating point A/cm^2 : Inport  Port=3  LatchInput=off
  Cell Gross Power Gen W/cm^2 : simulink3/Math/Dot Product
  Polarization Curve : Subsystem
      settings: RTWFcnNameOpts=Auto  RTWFileNameOpts=Auto
  Stack Gross Power Gen W1 : simulink3/Math/Dot Product
  stack area cm^2 : Constant  Value=fc_cell_area*fc_cell_num
  Cell Voltage : Outport  Port=1
  Stack Gross  Power Gen : Outport  Port=2
  wires:
  Cell Gross Power Gen W/cm^2/1 -> Stack Gross Power Gen W1/1
  stack area cm^2/1 -> Stack Gross Power Gen W1/2
  Stack Gross Power Gen W1/1 -> Stack Gross  Power Gen/1
  fc cell current density operating point A/cm^2/1 -> Cell Gross Power Gen W/cm^2/2, Polarization Curve/3(current)
  Fuel Cell  Stack Temperature/1 -> Polarization Curve/1(temperature)
  Average Partial Pressure Oxygen/1 -> Polarization Curve/2(po2)
  Polarization Curve/1(cell voltage) -> Cell Gross Power Gen W/cm^2/1, Cell Voltage/1

== system fc_vt_lib/Time Step ==
  Clock : Clock
      settings: DisplayTime=off  Decimation=10
  Memory : Memory  X0=-0.1  InheritSampleTime=off
      settings: RTWStateStorageClass=Auto
  Sum : Sum  Inputs=|+-  SaturateOnIntegerOverflow=on
  Out1 : Outport  Port=1
  wires:
  Clock/1 -> Sum/1, Memory/1
  Sum/1 -> Out1/1
  Memory/1 -> Sum/2
